simulink model "SingleTrack"  (R2019b)
settings: Solver=ode1  StartTime=0  StopTime=250  FixedStep=1.0000000000000000e-003  RelTol=1e-3
InitFcn:
  | sampleTime = str2double(get_param(bdroot, 'FixedStep'));
undefined symbols (not defined in the file or in its folder): AccPedalPos, BrakePedalPos, BrakeSwitch, DiscIntNeverNeededParam, DYNA4, EngSpd, IgnitionSwitch, InitialGear, InitialSpeed, IntendedEngTrq, LeftIndicator, MainBrakePress, MaxGear, MDL, MinGear, RefAcc, RefLane, RefLatPos, RefPath, RefPathCurv, RefSpd, RefSpdPreview, RefSpdRetrospect, RightIndicator, SteeringWheelAng, SteeringWheelTrq, UserDefinedRefValue, vm_const
libraries: UtilitiesLibrary x31, simulink x18, WheelSystemModules x13, LongitudinalControllerModules x13, LateralControllerModules x7, AnimationBusselectorModules x5, EnvironmentModules x5, BasicEngineControlModules x5, MiscellaneousControlModules x5, Animation3Modules x4, AuxiliariesModules x4, ReducedTireModules x4
(part 20 of 32)

== system SingleTrack/Vehicle/WheelSystem/FrontLeftWheelSystem/Tire ==
  fromCTRL : Inport
  fromChassis : Inport  Port=2
  fromWheel : Inport  Port=3
  Contact : WheelSystemModules/Contact  Tag=vedynaContactMask  local_comp_inst=1  system_comp_inst=1  sample_time=-1
  DynaComponentInfo : Subsystem  Tag=DynaComponentInfo
      mask init:
      | data= get_param(gcb, 'UserData');
      settings: OpenFcn=DYNA4.ModelHandling.Component.ShowEditComponentInformationDialog(gcb);
      mask Display: disp(['Type = ', data.type, '\nGroup = ', data.group, '\nName = ', data.name])
  Ground{1..3,5} (4 alike) : Ground
  InputFromCTRL : Subsystem  Tag=TESIS DYNAware Interface Block  mask{NeedsUpdate=off, SignalInfo=|}
      mask SignalInfo=|
      | {
      |   "Version": "4.6",
      |   "MuxedOutputBusName": "output",
      |   "MuxedInputBusName": "fromCTRL",
      |   "MuxedInputSelected": true,
      |   "MuxedOutputSelected": false,
      |   "SignalData": [
      |     {
      |       "initialValue": "0.0",
      |       "name": "AddRoadElev[m]",
      |       "comment": "",
      |       "minString": "",
      |       "maxString": "",
      |       "width": 1,
      |       "dataType": 0,
      |       "signalType": 0,
      |       "createSignal": false,
      |       "outputName": "AddRoadElev[m]",
      |       "generateSignalAccessBlock": false,
      |       "accessId": "$(parentId).$(blockName).$(outputName)"
      |     },
      |     {
      |       "initialValue": "0.0",
      |       "name": "RoadFrictionScaling[0_2]",
      |       "comment": "",
      |       "minString": "",
      |       "maxString": "",
      |       "width": 1,
      |       "dataType": 0,
      |       "signalType": 0,
      |       "createSignal": false,
      |       "outputName": "RoadFrictionScaling[0_2]",
      |       "generateSignalAccessBlock": false,
      |       "accessId": "$(parentId).$(blockName).$(outputName)"
      |     },
      |     {
      |       "initialValue": "0.0",
      |       "name": "AddLongRoadSlope[-]",
      |       "comment": "",
      |       "minString": "",
      |       "maxString": "",
      |       "width": 1,
      |       "dataType": 0,
      |       "signalType": 0,
      |       "createSignal": false,
      |       "outputName": "AddLongRoadSlope[-]",
      |       "generateSignalAccessBlock": false,
      |       "accessId": "$(parentId).$(blockName).$(outputName)"
      |     },
      |     {
      |       "initialValue": "0.0",
      |       "name": "AddLatRoadSlope[-]",
      |       "comment": "",
      |       "minString": "",
      |       "maxString": "",
      |       "width": 1,
      |       "dataType": 0,
      |       "signalType": 0,
      |       "createSignal": false,
      |       "outputName": "AddLatRoadSlope[-]",
      |       "generateSignalAccessBlock": false,
      |       "accessId": "$(parentId).$(blockName).$(outputName)"
      |     },
      |     {
      |       "initialValue": "0.0",
      |       "name": "LocalRoadSysSwitch[0;1]",
      |       "comment": "",
      |       "minString": "",
      |       "maxString": "",
      |       "width": 1,
      |       "dataType": 0,
      |       "signalType": 0,
      |       "createSignal": false,
      |       "outputName": "LocalRoadSysSwitch[0;1]",
      |       "generateSignalAccessBlock": false,
      |       "accessId": "$(parentId).$(blockName).$(outputName)"
      |     }
      |   ]
      | }
      mask prompts: NeedsUpdate "Specify, if subsystem content needs to be updated"; SignalInfo "Signal Info (json)"
      mask help: DYNA4 Interface Block Version 4.6
      mask init:
      | blockName = get_param(gcbh, 'Name');
      | parentId = DYNA4.ModelHandling.AccessID.getFromHierarchy(gcbh);
      | TD.InterfaceBlock.ModelCallbacks.GenerateContent(gcb);
      settings: DeleteFcn=TD.InterfaceBlock.ModelCallbacks.CloseGUI( gcbh );  NameChangeFcn=TD.InterfaceBlock.ModelCallbacks.BlockRenamedHandler(gcbh);  OpenFcn=TD.InterfaceBlock.ModelCallbacks.OpenGUI( gcbh );  CloseFcn=TD.InterfaceBlock.ModelCallbacks.CloseGUI( gcbh );
      mask Display:
      | image('InterfaceBlock.png','center');
      | port_label('input',1, 'fromCTRL');
      | port_label('output',1, 'AddRoadElev[m]');
      | port_label('output',2, 'RoadFrictionScaling[0_2]');
      | port_label('output',3, 'AddLongRoadSlope[-]');
      | port_label('output',4, 'AddLatRoadSlope[-]');
      | port_label('output',5, 'LocalRoadSysSwitch[0;1]');
  InputFromChassis : Subsystem  Tag=TESIS DYNAware Interface Block  mask{NeedsUpdate=off, SignalInfo=|}
      mask SignalInfo=|
      | {
      |   "Version": "4.6",
      |   "MuxedOutputBusName": "output",
      |   "MuxedInputBusName": "fromChassis",
      |   "MuxedInputSelected": true,
      |   "MuxedOutputSelected": false,
      |   "SignalData": [
      |     {
      |       "initialValue": "0.0",
      |       "name": "VehicleBody.PosAxleSys(WorldSys)",
      |       "comment": "",
      |       "minString": "",
      |       "maxString": "",
      |       "width": -1,
      |       "dataType": 0,
      |       "signalType": 0,
      |       "createSignal": false,
      |       "outputName": "PosAxleSys(WorldSys)",
      |       "generateSignalAccessBlock": false,
      |       "accessId": "$(parentId).$(blockName).$(outputName)"
      |     },
      |     {
      |       "initialValue": "0.0",
      |       "name": "VehicleBody.RotMatrix(WorldSys)[-]",
      |       "comment": "",
      |       "minString": "",
      |       "maxString": "",
      |       "width": 9,
      |       "dataType": 0,
      |       "signalType": 0,
      |       "createSignal": false,
      |       "outputName": "RotMatrix(WorldSys)[-]",
      |       "generateSignalAccessBlock": false,
      |       "accessId": "$(parentId).$(blockName).$(outputName)"
      |     },
      |     {
      |       "initialValue": "0.0",
      |       "name": "WheelSystem.WheelRotAxis(VehSys)[-]",
      |       "comment": "",
      |       "minString": "",
      |       "maxString": "",
      |       "width": 3,
      |       "dataType": 0,
      |       "signalType": 0,
      |       "createSignal": false,
      |       "outputName": "WheelRotAxis(VehSys)[-]",
      |       "generateSignalAccessBlock": false,
      |       "accessId": "$(parentId).$(blockName).$(outputName)"
      |     },
      |     {
      |       "initialValue": "0.0",
      |       "name": "WheelSystem.TirePos(AxleSys)[m]",
      |       "comment": "",
      |       "minString": "",
      |       "maxString": "",
      |       "width": -1,
      |       "dataType": 0,
      |       "signalType": 0,
      |       "createSignal": false,
      |       "outputName": "TirePos(AxleSys)[m]",
      |       "generateSignalAccessBlock": false,
      |       "accessId": "$(parentId).$(blockName).$(outputName)"
      |     },
      |     {
      |       "initialValue": "0.0",
      |       "name": "WheelSystem.TireVel_wrt_WorldSys(VehSys)[m/s]",
      |       "comment": "",
      |       "minString": "",
      |       "maxString": "",
      |       "width": 3,
      |       "dataType": 0,
      |       "signalType": 0,
      |       "createSignal": false,
      |       "outputName": "TireVel_wrt_WorldSys(VehSys)[m/s]",
      |       "generateSignalAccessBlock": false,
      |       "accessId": "$(parentId).$(blockName).$(outputName)"
      |     },
      |     {
      |       "initialValue": "0.0",
      |       "name": "WheelSystem.WheelRotVel_wrt_WorldSys(VehSys)[rad/s]",
      |       "comment": "",
      |       "minString": "",
      |       "maxString": "",
      |       "width": 3,
      |       "dataType": 0,
      |       "signalType": 0,
      |       "createSignal": false,
      |       "outputName": "WheelRotVel_wrt_WorldSys(VehSys)[rad/s]",
      |       "generateSignalAccessBlock": false,
      |       "accessId": "$(parentId).$(blockName).$(outputName)"
      |     },
      |     {
      |       "initialValue": "0.0",
      |       "name": "VehicleBody.Vel_wrt_WorldSys(VehSys)[m/s]",
      |       "comment": "",
      |       "minString": "",
      |       "maxString": "",
      |       "width": 3,
      |       "dataType": 0,
      |       "signalType": 0,
      |       "createSignal": false,
      |       "outputName": "Vel_wrt_WorldSys(VehSys)[m/s]",
      |       "generateSignalAccessBlock": false,
      |       "accessId": "$(parentId).$(blockName).$(outputName)"
      |     },
      |     {
      |       "initialValue": "0.0",
      |       "name": "WheelSystem.WheelRotMatrix(WorldSys)[-]",
      |       "comment": "",
      |       "minString": "",
      |       "maxString": "",
      |       "width": 9,
      |       "dataType": 0,
      |       "signalType": 0,
      |       "createSignal": false,
      |       "outputName": "WheelRotMatrix(WorldSys)[-]",
      |       "generateSignalAccessBlock": false,
      |       "accessId": "$(parentId).$(blockName).$(outputName)"
      |     },
      |     {
      |       "initialValue": "0.0",
      |       "name": "WheelSystem.TireDefl[m]",
      |       "comment": "",
      |       "minString": "",
      |       "maxString": "",
      |       "width": 1,
      |       "dataType": 0,
      |       "signalType": 0,
      |       "createSignal": false,
      |       "outputName": "TireDefl[m]",
      |       "generateSignalAccessBlock": false,
      |       "accessId": "$(parentId).$(blockName).$(outputName)"
      |     }
      |   ]
      | }
      mask prompts: NeedsUpdate "Specify, if subsystem content needs to be updated"; SignalInfo "Signal Info (json)"
      mask help: DYNA4 Interface Block Version 4.6
      mask init:
      | blockName = get_param(gcbh, 'Name');
      | parentId = DYNA4.ModelHandling.AccessID.getFromHierarchy(gcbh);
      | TD.InterfaceBlock.ModelCallbacks.GenerateContent(gcb);
      settings: DeleteFcn=TD.InterfaceBlock.ModelCallbacks.CloseGUI( gcbh );  NameChangeFcn=TD.InterfaceBlock.ModelCallbacks.BlockRenamedHandler(gcbh);  OpenFcn=TD.InterfaceBlock.ModelCallbacks.OpenGUI( gcbh );  CloseFcn=TD.InterfaceBlock.ModelCallbacks.CloseGUI( gcbh );
      mask Display:
      | image('InterfaceBlock.png','center');
      | port_label('input',1, 'fromChassis');
      | port_label('output',1, 'PosAxleSys(WorldSys)');
      | port_label('output',2, 'RotMatrix(WorldSys)[-]');
      | port_label('output',3, 'WheelRotAxis(VehSys)[-]');
      | port_label('output',4, 'TirePos(AxleSys)[m]');
      | port_label('output',5, 'TireVel_wrt_WorldSys(VehSys)[m/s]');
      | port_label('output',6, 'WheelRotVel_wrt_WorldSys(VehSys)[rad/s]');
      | port_label('output',7, 'Vel_wrt_WorldSys(VehSys)[m/s]');
      | port_label('output',8, 'WheelRotMatrix(WorldSys)[-]');
      | port_label('output',9, 'TireDefl[m]');
  InputFromWheel : Subsystem  Tag=TESIS DYNAware Interface Block  mask{NeedsUpdate=off, SignalInfo=|}
      mask SignalInfo=|
      | {
      |   "Version": "4.6",
      |   "MuxedOutputBusName": "fromWheel",
      |   "MuxedInputBusName": "fromWheel",
      |   "MuxedInputSelected": true,
      |   "MuxedOutputSelected": false,
      |   "SignalData": [
      |     {
      |       "initialValue": "0.0",
      |       "name": "RotSpd[rad/s]",
      |       "comment": "",
      |       "minString": "",
      |       "maxString": "",
      |       "width": 1,
      |       "dataType": 0,
      |       "signalType": 0,
      |       "createSignal": false,
      |       "outputName": "RotSpd[rad/s]",
      |       "generateSignalAccessBlock": false,
      |       "accessId": "$(parentId).$(blockName).$(outputName)"
      |     },
      |     {
      |       "initialValue": "0.0",
      |       "name": "BlockingState[0;1]",
      |       "comment": "",
      |       "minString": "",
      |       "maxString": "",
      |       "width": 1,
      |       "dataType": 0,
      |       "signalType": 0,
      |       "createSignal": false,
      |       "outputName": "BlockingState[0;1]",
      |       "generateSignalAccessBlock": false,
      |       "accessId": "$(parentId).$(blockName).$(outputName)"
      |     }
      |   ]
      | }
      mask prompts: NeedsUpdate "Specify, if subsystem content needs to be updated"; SignalInfo "Signal Info (json)"
      mask help: DYNA4 Interface Block Version 4.6
      mask init:
      | blockName = get_param(gcbh, 'Name');
      | parentId = DYNA4.ModelHandling.AccessID.getFromHierarchy(gcbh);
      | TD.InterfaceBlock.ModelCallbacks.GenerateContent(gcb);
      settings: DeleteFcn=TD.InterfaceBlock.ModelCallbacks.CloseGUI( gcbh );  NameChangeFcn=TD.InterfaceBlock.ModelCallbacks.BlockRenamedHandler(gcbh);  OpenFcn=TD.InterfaceBlock.ModelCallbacks.OpenGUI( gcbh );  CloseFcn=TD.InterfaceBlock.ModelCallbacks.CloseGUI( gcbh );
      mask Display:
      | image('InterfaceBlock.png','center');
      | port_label('input',1, 'fromWheel');
      | port_label('output',1, 'RotSpd[rad/s]');
      | port_label('output',2, 'BlockingState[0;1]');
  Memory1 : Memory  InheritSampleTime=on
  TabledTireForces : ReducedTireModules/TabledTireForces  Tag=vedynaTabledConsumptionMask  DATA_NODE=MDL.Vehicle.WheelSystem.FrontLeft.Tire.TabledTireForces  UnloadedRadius=MDL.Vehicle.WheelSystem.FrontLeft.Tire.TabledTireForces.UnloadedRadius  WidthToRadiusRatio=MDL.Vehicle.WheelSystem.FrontLeft.Tire.TabledTireForces.WidthToRadiusRatio  HeightToRadiusRatio=MDL.Vehicle.WheelSystem.FrontLeft.Tire.TabledTireForces.HeightToRadiusRatio  RefLoad=MDL.Vehicle.WheelSystem.FrontLeft.Tire.TabledTireForces.RefLoad  LongFrcCurve=MDL.Vehicle.WheelSystem.FrontLeft.Tire.TabledTireForces.LongFrcCurve  LatFrcCurve=MDL.Vehicle.WheelSystem.FrontLeft.Tire.TabledTireForces.LatFrcCurve  RollResistance=MDL.Vehicle.WheelSystem.FrontLeft.Tire.TabledTireForces.RollResistCoeff  VertStiff=MDL.Vehicle.WheelSystem.FrontLeft.Tire.TabledTireForces.VertStiff
  Tire Output : Subsystem  Tag=TESIS DYNAware Interface Block  mask{NeedsUpdate=off, SignalInfo=|}
      mask SignalInfo=|
      | {
      |   "Version": "4.6",
      |   "MuxedOutputBusName": "Tire",
      |   "MuxedInputBusName": "input",
      |   "MuxedInputSelected": false,
      |   "MuxedOutputSelected": true,
      |   "SignalData": [
      |     {
      |       "initialValue": "0.0",
      |       "name": "ContactPointPos_wrt_WheelCenter(WorldSys)[m]",
      |       "comment": "",
      |       "minString": "",
      |       "maxString": "",
      |       "width": 3,
      |       "dataType": 0,
      |       "signalType": 0,
      |       "createSignal": false,
      |       "outputName": "ContactPointPos_wrt_WheelCenter(WorldSys)[m]",
      |       "generateSignalAccessBlock": false,
      |       "accessId": "$(parentId).$(blockName).$(outputName)"
      |     },
      |     {
      |       "initialValue": "0.0",
      |       "name": "CamberAng(ContactSys)[rad]",
      |       "comment": "",
      |       "minString": "",
      |       "maxString": "",
      |       "width": 1,
      |       "dataType": 0,
      |       "signalType": 0,
      |       "createSignal": false,
      |       "outputName": "CamberAng(ContactSys)[rad]",
      |       "generateSignalAccessBlock": false,
      |       "accessId": "$(parentId).$(blockName).$(outputName)"
      |     },
      |     {
      |       "initialValue": "0.0",
      |       "name": "TireDefl[m]",
      |       "comment": "",
      |       "minString": "",
      |       "maxString": "",
      |       "width": 1,
      |       "dataType": 0,
      |       "signalType": 0,
      |       "createSignal": false,
      |       "outputName": "TireDefl[m]",
      |       "generateSignalAccessBlock": false,
      |       "accessId": "$(parentId).$(blockName).$(outputName)"
      |     },
      |     {
      |       "initialValue": "0.0",
      |       "name": "TireDeflSpd[m/s]",
      |       "comment": "",
      |       "minString": "",
      |       "maxString": "",
      |       "width": 1,
      |       "dataType": 0,
      |       "signalType": 0,
      |       "createSignal": false,
      |       "outputName": "TireDeflSpd[m/s]",
      |       "generateSignalAccessBlock": false,
      |       "accessId": "$(parentId).$(blockName).$(outputName)"
      |     },
      |     {
      |       "initialValue": "0.0",
      |       "name": "LongSpd(ContactSys)[m/s]",
      |       "comment": "",
      |       "minString": "",
      |       "maxString": "",
      |       "width": 1,
      |       "dataType": 0,
      |       "signalType": 0,
      |       "createSignal": false,
      |       "outputName": "LongSpd(ContactSys)[m/s]",
      |       "generateSignalAccessBlock": false,
      |       "accessId": "$(parentId).$(blockName).$(outputName)"
      |     },
      |     {
      |       "initialValue": "0.0",
      |       "name": "LatSpd(ContactSys)[m/s]",
      |       "comment": "",
      |       "minString": "",
      |       "maxString": "",
      |       "width": 1,
      |       "dataType": 0,
      |       "signalType": 0,
      |       "createSignal": false,
      |       "outputName": "LatSpd(ContactSys)[m/s]",
      |       "generateSignalAccessBlock": false,
      |       "accessId": "$(parentId).$(blockName).$(outputName)"
      |     },
      |     {
      |       "initialValue": "0.0",
      |       "name": "BoreSpd(ContactSys)[rad/s]",
      |       "comment": "",
      |       "minString": "",
      |       "maxString": "",
      |       "width": 1,
      |       "dataType": 0,
      |       "signalType": 0,
      |       "createSignal": false,
      |       "outputName": "BoreSpd(ContactSys)[rad/s]",
      |       "generateSignalAccessBlock": false,
      |       "accessId": "$(parentId).$(blockName).$(outputName)"
      |     },
      |     {
      |       "initialValue": "0.0",
      |       "name": "LongFrcLeverArm_wrt_WheelRotAxis[m]",
      |       "comment": "",
      |       "minString": "",
      |       "maxString": "",
      |       "width": 1,
      |       "dataType": 0,
      |       "signalType": 0,
      |       "createSignal": false,
      |       "outputName": "LongFrcLeverArm_wrt_WheelRotAxis[m]",
      |       "generateSignalAccessBlock": false,
      |       "accessId": "$(parentId).$(blockName).$(outputName)"
      |     },
      |     {
      |       "initialValue": "0.0",
      |       "name": "LongUnitVector(WorldSys)[-]",
      |       "comment": "",
      |       "minString": "",
      |       "maxString": "",
      |       "width": 3,
      |       "dataType": 0,
      |       "signalType": 0,
      |       "createSignal": false,
      |       "outputName": "LongUnitVector(WorldSys)[-]",
      |       "generateSignalAccessBlock": false,
      |       "accessId": "$(parentId).$(blockName).$(outputName)"
      |     },
      |     {
      |       "initialValue": "0.0",
      |       "name": "LatUnitVector(WorldSys)[-]",
      |       "comment": "",
      |       "minString": "",
      |       "maxString": "",
      |       "width": 3,
      |       "dataType": 0,
      |       "signalType": 0,
      |       "createSignal": false,
      |       "outputName": "LatUnitVector(WorldSys)[-]",
      |       "generateSignalAccessBlock": false,
      |       "accessId": "$(parentId).$(blockName).$(outputName)"
      |     },
      |     {
      |       "initialValue": "0.0",
      |       "name": "RoadNormalVector(WorldSys)[-]",
      |       "comment": "",
      |       "minString": "",
      |       "maxString": "",
      |       "width": 3,
      |       "dataType": 0,
      |       "signalType": 0,
      |       "createSignal": false,
      |       "outputName": "RoadNormalVector(WorldSys)[-]",
      |       "generateSignalAccessBlock": false,
      |       "accessId": "$(parentId).$(blockName).$(outputName)"
      |     },
      |     {
      |       "initialValue": "0.0",
      |       "name": "RoadType[-]",
      |       "comment": "",
      |       "minString": "",
      |       "maxString": "",
      |       "width": 1,
      |       "dataType": 0,
      |       "signalType": 0,
      |       "createSignal": false,
      |       "outputName": "RoadType[-]",
      |       "generateSignalAccessBlock": false,
      |       "accessId": "$(parentId).$(blockName).$(outputName)"
      |     },
      |     {
      |       "initialValue": "0.0",
      |       "name": "RoadFrictionScalingCoeff[-]",
      |       "comment": "",
      |       "minString": "",
      |       "maxString": "",
      |       "width": 1,
      |       "dataType": 0,
      |       "signalType": 0,
      |       "createSignal": false,
      |       "outputName": "RoadFrictionScalingCoeff[-]",
      |       "generateSignalAccessBlock": false,
      |       "accessId": "$(parentId).$(blockName).$(outputName)"
      |     },
      |     {
      |       "initialValue": "0.0",
      |       "name": "ContactPointPos(WorldSys)[m]",
      |       "comment": "",
      |       "minString": "",
      |       "maxString": "",
      |       "width": 3,
      |       "dataType": 0,
      |       "signalType": 0,
      |       "createSignal": false,
      |       "outputName": "ContactPointPos(WorldSys)[m]",
      |       "generateSignalAccessBlock": false,
      |       "accessId": "$(parentId).$(blockName).$(outputName)"
      |     },
      |     {
      |       "initialValue": "0.0",
      |       "name": "RoadSlope(WorldSys)[-]",
      |       "comment": "",
      |       "minString": "",
      |       "maxString": "",
      |       "width": 1,
      |       "dataType": 0,
      |       "signalType": 0,
      |       "createSignal": false,
      |       "outputName": "RoadSlope(WorldSys)[-]",
      |       "generateSignalAccessBlock": false,
      |       "accessId": "$(parentId).$(blockName).$(outputName)"
      |     },
      |     {
      |       "initialValue": "0.0",
      |       "name": "RoadIncl(WorldSys)[-]",
      |       "comment": "",
      |       "minString": "",
      |       "maxString": "",
      |       "width": 1,
      |       "dataType": 0,
      |       "signalType": 0,
      |       "createSignal": false,
      |       "outputName": "RoadIncl(WorldSys)[-]",
      |       "generateSignalAccessBlock": false,
      |       "accessId": "$(parentId).$(blockName).$(outputName)"
      |     },
      |     {
      |       "initialValue": "0.0",
      |       "name": "LocalContactPoints(WorldSys)[m]",
      |       "comment": "",
      |       "minString": "",
      |       "maxString": "",
      |       "width": 12,
      |       "dataType": 0,
      |       "signalType": 0,
      |       "createSignal": false,
      |       "outputName": "LocalContactPoints(WorldSys)[m]",
      |       "generateSignalAccessBlock": false,
      |       "accessId": "$(parentId).$(blockName).$(outputName)"
      |     },
      |     {
      |       "initialValue": "0.0",
      |       "name": "NumberOfLocalContactPoints[-]",
      |       "comment": "",
      |       "minString": "",
      |       "maxString": "",
      |       "width": 1,
      |       "dataType": 0,
      |       "signalType": 0,
      |       "createSignal": false,
      |       "outputName": "NumberOfLocalContactPoints[-]",
      |       "generateSignalAccessBlock": false,
      |       "accessId": "$(parentId).$(blockName).$(outputName)"
      |     },
      |     {
      |       "initialValue": "0.0",
      |       "name": "WheelCenterFrc(VehSys)[N]",
      |       "comment": "",
      |       "minString": "",
      |       "maxString": "",
      |       "width": 3,
      |       "dataType": 0,
      |       "signalType": 0,
      |       "createSignal": false,
      |       "outputName": "WheelCenterFrc(VehSys)[N]",
      |       "generateSignalAccessBlock": false,
      |       "accessId": "$(parentId).$(blockName).$(outputName)"
      |     },
      |     {
      |       "initialValue": "0.0",
      |       "name": "CircumferentialTrq_wrt_WheelRotAxis[Nm]",
      |       "comment": "",
      |       "minString": "",
      |       "maxString": "",
      |       "width": 1,
      |       "dataType": 0,
      |       "signalType": 0,
      |       "createSignal": false,
      |       "outputName": "CircumferentialTrq_wrt_WheelRotAxis[Nm]",
      |       "generateSignalAccessBlock": false,
      |       "accessId": "$(parentId).$(blockName).$(outputName)"
      |     },
      |     {
      |       "initialValue": "0.0",
      |       "name": "MaxRollResistTrq[Nm]",
      |       "comment": "",
      |       "minString": "",
      |       "maxString": "",
      |       "width": 1,
      |       "dataType": 0,
      |       "signalType": 0,
      |       "createSignal": false,
      |       "outputName": "MaxRollResistTrq[Nm]",
      |       "generateSignalAccessBlock": false,
      |       "accessId": "$(parentId).$(blockName).$(outputName)"
      |     },
      |     {
      |       "initialValue": "0.0",
      |       "name": "VertStiff[N/m]",
      |       "comment": "",
      |       "minString": "",
      |       "maxString": "",
      |       "width": 1,
      |       "dataType": 0,
      |       "signalType": 0,
      |       "createSignal": false,
      |       "outputName": "VertStiff[N/m]",
      |       "generateSignalAccessBlock": false,
      |       "accessId": "$(parentId).$(blockName).$(outputName)"
      |     },
      |     {
      |       "initialValue": "0.0",
      |       "name": "UnloadedRadius[m]",
      |       "comment": "",
      |       "minString": "",
      |       "maxString": "",
      |       "width": 1,
      |       "dataType": 0,
      |       "signalType": 0,
      |       "createSignal": false,
      |       "outputName": "UnloadedRadius[m]",
      |       "generateSignalAccessBlock": false,
      |       "accessId": "$(parentId).$(blockName).$(outputName)"
      |     },
      |     {
      |       "initialValue": "0.0",
      |       "name": "RimRadius[m]",
      |       "comment": "",
      |       "minString": "",
      |       "maxString": "",
      |       "width": 1,
      |       "dataType": 0,
      |       "signalType": 0,
      |       "createSignal": false,
      |       "outputName": "RimRadius[m]",
      |       "generateSignalAccessBlock": false,
      |       "accessId": "$(parentId).$(blockName).$(outputName)"
      |     },
      |     {
      |       "initialValue": "0.0",
      |       "name": "Width[m]",
      |       "comment": "",
      |       "minString": "",
      |       "maxString": "",
      |       "width": 1,
      |       "dataType": 0,
      |       "signalType": 0,
      |       "createSignal": false,
      |       "outputName": "Width[m]",
      |       "generateSignalAccessBlock": false,
      |       "accessId": "$(parentId).$(blockName).$(outputName)"
      |     },
      |     {
      |       "initialValue": "0.0",
      |       "name": "ContactPointFrc(ContactSys)[N]",
      |       "comment": "",
      |       "minString": "",
      |       "maxString": "",
      |       "width": 3,
      |       "dataType": 0,
      |       "signalType": 0,
      |       "createSignal": false,
      |       "outputName": "ContactPointFrc(ContactSys)[N]",
      |       "generateSignalAccessBlock": false,
      |       "accessId": "$(parentId).$(blockName).$(outputName)"
      |     },
      |     {
      |       "initialValue": "0.0",
      |       "name": "ContactPointTrq(ContactSys)[N]",
      |       "comment": "",
      |       "minString": "",
      |       "maxString": "",
      |       "width": 3,
      |       "dataType": 0,
      |       "signalType": 0,
      |       "createSignal": false,
      |       "outputName": "ContactPointTrq(ContactSys)[N]",
      |       "generateSignalAccessBlock": false,
      |       "accessId": "$(parentId).$(blockName).$(outputName)"
      |     },
      |     {
      |       "initialValue": "0.0",
      |       "name": "CorneringStiff[N]",
      |       "comment": "",
      |       "minString": "",
      |       "maxString": "",
      |       "width": 1,
      |       "dataType": 0,
      |       "signalType": 0,
      |       "createSignal": false,
      |       "outputName": "CorneringStiff[N]",
      |       "generateSignalAccessBlock": false,
      |       "accessId": "$(parentId).$(blockName).$(outputName)"
      |     },
      |     {
      |       "initialValue": "0.0",
      |       "name": "DynamicRadius[m]",
      |       "comment": "",
      |       "minString": "",
      |       "maxString": "",
      |       "width": 1,
      |       "dataType": 0,
      |       "signalType": 0,
      |       "createSignal": false,
      |       "outputName": "DynamicRadius[m]",
      |       "generateSignalAccessBlock": false,
      |       "accessId": "$(parentId).$(blockName).$(outputName)"
      |     },
      |     {
      |       "initialValue": "0.0",
      |       "name": "ContactPatchLength[m]",
      |       "comment": "",
      |       "minString": "",
      |       "maxString": "",
      |       "width": 1,
      |       "dataType": 0,
      |       "signalType": 0,
      |       "createSignal": false,
      |       "outputName": "ContactPatchLength[m]",
      |       "generateSignalAccessBlock": false,
      |       "accessId": "$(parentId).$(blockName).$(outputName)"
      |     },
      |     {
      |       "initialValue": "0.0",
      |       "name": "ContactPatchWidth[m]",
      |       "comment": "",
      |       "minString": "",
      |       "maxString": "",
      |       "width": 1,
      |       "dataType": 0,
      |       "signalType": 0,
      |       "createSignal": false,
      |       "outputName": "ContactPatchWidth[m]",
      |       "generateSignalAccessBlock": false,
      |       "accessId": "$(parentId).$(blockName).$(outputName)"
      |     }
      |   ]
      | }
      mask prompts: NeedsUpdate "Specify, if subsystem content needs to be updated"; SignalInfo "Signal Info (json)"
      mask help: DYNA4 Interface Block Version 4.6
      mask init:
      | blockName = get_param(gcbh, 'Name');
      | parentId = DYNA4.ModelHandling.AccessID.getFromHierarchy(gcbh);
      | TD.InterfaceBlock.ModelCallbacks.GenerateContent(gcb);
      settings: DeleteFcn=TD.InterfaceBlock.ModelCallbacks.CloseGUI( gcbh );  NameChangeFcn=TD.InterfaceBlock.ModelCallbacks.BlockRenamedHandler(gcbh);  OpenFcn=TD.InterfaceBlock.ModelCallbacks.OpenGUI( gcbh );  CloseFcn=TD.InterfaceBlock.ModelCallbacks.CloseGUI( gcbh );
      mask Display:
      | image('InterfaceBlock.png','center');
      | port_label('input',1, 'ContactPointPos_wrt_WheelCenter(WorldSys)[m]');
      | port_label('input',2, 'CamberAng(ContactSys)[rad]');
      | port_label('input',3, 'TireDefl[m]');
      | port_label('input',4, 'TireDeflSpd[m/s]');
      | port_label('input',5, 'LongSpd(ContactSys)[m/s]');
      | port_label('input',6, 'LatSpd(ContactSys)[m/s]');
      | port_label('input',7, 'BoreSpd(ContactSys)[rad/s]');
      | port_label('input',8, 'LongFrcLeverArm_wrt_WheelRotAxis[m]');
      | port_label('input',9, 'LongUnitVector(WorldSys)[-]');
      | port_label('input',10, 'LatUnitVector(WorldSys)[-]');
      | port_label('input',11, 'RoadNormalVector(WorldSys)[-]');
      | port_label('input',12, 'RoadType[-]');
      | port_label('input',13, 'RoadFrictionScalingCoeff[-]');
      | port_label('input',14, 'ContactPointPos(WorldSys)[m]');
      | port_label('input',15, 'RoadSlope(WorldSys)[-]');
      | port_label('input',16, 'RoadIncl(WorldSys)[-]');
      | port_label('input',17, 'LocalContactPoints(WorldSys)[m]');
      | port_label('input',18, 'NumberOfLocalContactPoints[-]');
      | port_label('input',19, 'WheelCenterFrc(VehSys)[N]');
      | port_label('input',20, 'CircumferentialTrq_wrt_WheelRotAxis[Nm]');
      | port_label('input',21, 'MaxRollResistTrq[Nm]');
      | port_label('input',22, 'VertStiff[N/m]');
      | port_label('input',23, 'UnloadedRadius[m]');
      | port_label('input',24, 'RimRadius[m]');
      | port_label('input',25, 'Width[m]');
      | port_label('input',26, 'ContactPointFrc(ContactSys)[N]');
      | port_label('input',27, 'ContactPointTrq(ContactSys)[N]');
      | port_label('input',28, 'CorneringStiff[N]');
      | port_label('input',29, 'DynamicRadius[m]');
      | port_label('input',30, 'ContactPatchLength[m]');
      | port_label('input',31, 'ContactPatchWidth[m]');
      | port_label('output',1, 'Tire');
  TraceMarker : UtilitiesLibrary/DYNA4 Trace Marker  Tag=DYNA4_TRACE_MARKER  SettingType=Standard  PrefixModelBlockID=on  PrefixRootSignalName=off  NamePattern='$(modelBlockID).$(rootSignalName)'
  Tire : Outport  VectorParamsAs1DForOutWhenUnconnected=off
  wires:
  InputFromWheel/1(RotSpd[rad/s]___UNIQUE_1) -> TabledTireForces/7, Contact/5
  TabledTireForces/9 -> Tire Output/28(CorneringStiff[N]___UNIQUE_1)
  TabledTireForces/8 -> Tire Output/26(ContactPointFrc(ContactSys)[N]___UNIQUE_1)
  Ground5/1 -> Contact/1
  Memory1/1 -> TabledTireForces/8
  TabledTireForces/7 -> Contact/4, Tire Output/25(Width[m]___UNIQUE_1)
  fromChassis/1 -> InputFromChassis/1(fromChassis)
  fromCTRL/1 -> InputFromCTRL/1(fromCTRL)
  InputFromCTRL/5(LocalRoadSysSwitch[0;1]___UNIQUE_1) -> Contact/16
  InputFromCTRL/4(AddLatRoadSlope[-]___UNIQUE_1) -> Contact/15
  InputFromCTRL/3(AddLongRoadSlope[-]___UNIQUE_1) -> Contact/14
  InputFromCTRL/2(RoadFrictionScaling[0_2]___UNIQUE_1) -> Contact/13
  InputFromCTRL/1(AddRoadElev[m]___UNIQUE_1) -> Contact/12
  InputFromChassis/6(WheelRotVel_wrt_WorldSys(VehSys)[rad/s]___UNIQUE_1) -> Contact/11
  InputFromChassis/5(TireVel_wrt_WorldSys(VehSys)[m/s]___UNIQUE_1) -> Contact/10
  InputFromChassis/3(WheelRotAxis(VehSys)[-]___UNIQUE_1) -> Contact/8
  InputFromChassis/2(RotMatrix(WorldSys)[-]___UNIQUE_1) -> Contact/7, TabledTireForces/4
  InputFromChassis/1(PosAxleSys(WorldSys)___UNIQUE_1) -> Contact/6
  Contact/16 -> Tire Output/16(RoadIncl(WorldSys)[-]___UNIQUE_1)
  Contact/15 -> Tire Output/15(RoadSlope(WorldSys)[-]___UNIQUE_1)
  Contact/14 -> Tire Output/14(ContactPointPos(WorldSys)[m]___UNIQUE_1)
  Contact/13 -> Tire Output/13(RoadFrictionScalingCoeff[-]___UNIQUE_1)
  Contact/12 -> Tire Output/12(RoadType[-]___UNIQUE_1)
  Contact/11 -> Tire Output/11(RoadNormalVector(WorldSys)[-]___UNIQUE_1)
  Contact/10 -> Tire Output/10(LatUnitVector(WorldSys)[-]___UNIQUE_1)
  Contact/9 -> Tire Output/9(LongUnitVector(WorldSys)[-]___UNIQUE_1)
  Contact/8 -> Tire Output/8(LongFrcLeverArm_wrt_WheelRotAxis[m]___UNIQUE_1)
  Contact/7 -> Tire Output/7(BoreSpd(ContactSys)[rad/s]___UNIQUE_1)
  Contact/6 -> TabledTireForces/2, Tire Output/6(LatSpd(ContactSys)[m/s]___UNIQUE_1)
  Contact/5 -> TabledTireForces/1, Tire Output/5(LongSpd(ContactSys)[m/s]___UNIQUE_1)
  Contact/4 -> Tire Output/4(TireDeflSpd[m/s]___UNIQUE_1)
  Contact/3 -> Tire Output/3(TireDefl[m]___UNIQUE_1)
  Contact/2 -> Tire Output/2(CamberAng(ContactSys)[rad]___UNIQUE_1)
  Contact/1 -> Tire Output/1(ContactPointPos_wrt_WheelCenter(WorldSys)[m]___UNIQUE_1)
  Tire Output/1(Tire___UNIQUE_1) -> Tire/1, TraceMarker/1
  fromWheel/1 -> InputFromWheel/1(fromWheel)
  TabledTireForces/2 -> Tire Output/20(CircumferentialTrq_wrt_WheelRotAxis[Nm]___UNIQUE_1)
  TabledTireForces/4 -> Tire Output/22(VertStiff[N/m]___UNIQUE_1)
  TabledTireForces/6 -> Contact/3, Tire Output/24(RimRadius[m]___UNIQUE_1)
  TabledTireForces/3 -> Tire Output/21(MaxRollResistTrq[Nm]___UNIQUE_1)
  TabledTireForces/1 -> Tire Output/19(WheelCenterFrc(VehSys)[N]___UNIQUE_1)
  InputFromChassis/7(Vel_wrt_WorldSys(VehSys)[m/s]___UNIQUE_1) -> TabledTireForces/5
  InputFromChassis/8(WheelRotMatrix(WorldSys)[-]___UNIQUE_1) -> TabledTireForces/6
  InputFromWheel/2(BlockingState[0;1]___UNIQUE_1) -> Memory1/1
  TabledTireForces/5 -> Contact/2, Tire Output/23(UnloadedRadius[m]___UNIQUE_1), Tire Output/29(DynamicRadius[m]___UNIQUE_1)
  InputFromChassis/9(TireDefl[m]___UNIQUE_1) -> TabledTireForces/3
  Contact/17 -> Tire Output/17(LocalContactPoints(WorldSys)[m]___UNIQUE_1)
  Contact/18 -> Tire Output/18(NumberOfLocalContactPoints[-]___UNIQUE_1)
  Ground1/1 -> Tire Output/30(ContactPatchLength[m]___UNIQUE_1)
  Ground2/1 -> Tire Output/27(ContactPointTrq(ContactSys)[N]___UNIQUE_1)
  Ground3/1 -> Tire Output/31(ContactPatchWidth[m]___UNIQUE_1)
  InputFromChassis/4(TirePos(AxleSys)[m]___UNIQUE_1) -> Contact/9

== system SingleTrack/Vehicle/WheelSystem/FrontLeftWheelSystem/WheelOutput ==
  DriveBrakeTrq_wrt_WheelRotAxis(VehSys)[Nm]___UNIQUE_1 : Inport  Description=|  PortDimensions=[3]
      | <name>DriveBrakeTrq_wrt_WheelRotAxis(VehSys)[Nm]</name>
      | <comment></comment>
  RotSpd[rad/s]___UNIQUE_1 : Inport  Description=|  Port=2  PortDimensions=[1]
      | <name>RotSpd[rad/s]</name>
      | <comment></comment>
  RotAcc[rad/s**2]___UNIQUE_1 : Inport  Description=|  Port=3  PortDimensions=[1]
      | <name>RotAcc[rad/s**2]</name>
      | <comment></comment>
  BlockingState[0;1]___UNIQUE_1 : Inport  Description=|  Port=4  PortDimensions=[1]
      | <name>BlockingState[0;1]</name>
      | <comment></comment>
  RotAng[rad]___UNIQUE_1 : Inport  Description=|  Port=5  PortDimensions=[1]
      | <name>RotAng[rad]</name>
      | <comment></comment>
  BrakeTrqPressRatio[m**3]___UNIQUE_1 : Inport  Description=|  Port=6  PortDimensions=[1]
      | <name>BrakeTrqPressRatio[m**3]</name>
      | <comment></comment>
  RotAxisInrt[kg*m**2]___UNIQUE_1 : Inport  Description=|  Port=7  PortDimensions=[1]
      | <name>RotAxisInrt[kg*m**2]</name>
      | <comment></comment>
  TotalResistanceTorque[Nm]___UNIQUE_1 : Inport  Description=|  Port=8  PortDimensions=[1]
      | <name>TotalResistanceTorque[Nm]</name>
      | <comment></comment>
  KinematicWheelActiveFlag[0;1]___UNIQUE_1 : Inport  Description=|  Port=9  PortDimensions=[1]
      | <name>KinematicWheelActiveFlag[0;1]</name>
      | <comment></comment>
  VehBodyReplacementInrt[kg*m**2]___UNIQUE_1 : Inport  Description=|  Port=10  PortDimensions=[1]
      | <name>VehBodyReplacementInrt[kg*m**2]</name>
      | <comment></comment>
  __TDD__Wheel.BlockingState[0;1] : Demux  Outputs=[1]
  __TDD__Wheel.BrakeTrqPressRatio[m**3] : Demux  Outputs=[1]
  __TDD__Wheel.DriveBrakeTrq_wrt_WheelRotAxis(VehSys)[Nm] : Demux  Outputs=[3]
  __TDD__Wheel.KinematicWheelActiveFlag[0;1] : Demux  Outputs=[1]
  __TDD__Wheel.RotAcc[rad/s**2] : Demux  Outputs=[1]
  __TDD__Wheel.RotAng[rad] : Demux  Outputs=[1]
  __TDD__Wheel.RotAxisInrt[kg*m**2] : Demux  Outputs=[1]
  __TDD__Wheel.RotSpd[rad/s] : Demux  Outputs=[1]
  __TDD__Wheel.TotalResistanceTorque[Nm] : Demux  Outputs=[1]
  __TDD__Wheel.VehBodyReplacementInrt[kg*m**2] : Demux  Outputs=[1]
  __TDO__Wheel : BusCreator  Inputs=10
  Wheel___UNIQUE_1 : Outport  Description=|  PortDimensions=[12]  VectorParamsAs1DForOutWhenUnconnected=off
      | <name>DriveBrakeTrq_wrt_WheelRotAxis(VehSys)[Nm]</name>
      | <comment></comment>
  wires:
  __TDO__Wheel/1 -> Wheel___UNIQUE_1/1  "Wheel"
  __TDD__Wheel.VehBodyReplacementInrt[kg*m**2]/1 -> __TDO__Wheel/10  "VehBodyReplacementInrt[kg*m**2]"
  VehBodyReplacementInrt[kg*m**2]___UNIQUE_1/1 -> __TDD__Wheel.VehBodyReplacementInrt[kg*m**2]/1
  __TDD__Wheel.KinematicWheelActiveFlag[0;1]/1 -> __TDO__Wheel/9  "KinematicWheelActiveFlag[0;1]"
  KinematicWheelActiveFlag[0;1]___UNIQUE_1/1 -> __TDD__Wheel.KinematicWheelActiveFlag[0;1]/1
  __TDD__Wheel.TotalResistanceTorque[Nm]/1 -> __TDO__Wheel/8  "TotalResistanceTorque[Nm]"
  TotalResistanceTorque[Nm]___UNIQUE_1/1 -> __TDD__Wheel.TotalResistanceTorque[Nm]/1
  __TDD__Wheel.RotAxisInrt[kg*m**2]/1 -> __TDO__Wheel/7  "RotAxisInrt[kg*m**2]"
  RotAxisInrt[kg*m**2]___UNIQUE_1/1 -> __TDD__Wheel.RotAxisInrt[kg*m**2]/1
  __TDD__Wheel.BrakeTrqPressRatio[m**3]/1 -> __TDO__Wheel/6  "BrakeTrqPressRatio[m**3]"
  BrakeTrqPressRatio[m**3]___UNIQUE_1/1 -> __TDD__Wheel.BrakeTrqPressRatio[m**3]/1
  __TDD__Wheel.RotAng[rad]/1 -> __TDO__Wheel/5  "RotAng[rad]"
  RotAng[rad]___UNIQUE_1/1 -> __TDD__Wheel.RotAng[rad]/1
  __TDD__Wheel.BlockingState[0;1]/1 -> __TDO__Wheel/4  "BlockingState[0;1]"
  BlockingState[0;1]___UNIQUE_1/1 -> __TDD__Wheel.BlockingState[0;1]/1
  __TDD__Wheel.RotAcc[rad/s**2]/1 -> __TDO__Wheel/3  "RotAcc[rad/s**2]"
  RotAcc[rad/s**2]___UNIQUE_1/1 -> __TDD__Wheel.RotAcc[rad/s**2]/1
  __TDD__Wheel.RotSpd[rad/s]/1 -> __TDO__Wheel/2  "RotSpd[rad/s]"
  RotSpd[rad/s]___UNIQUE_1/1 -> __TDD__Wheel.RotSpd[rad/s]/1
  __TDD__Wheel.DriveBrakeTrq_wrt_WheelRotAxis(VehSys)[Nm]/1 -> __TDO__Wheel/1  "DriveBrakeTrq_wrt_WheelRotAxis(VehSys)[Nm]"
  DriveBrakeTrq_wrt_WheelRotAxis(VehSys)[Nm]___UNIQUE_1/1 -> __TDD__Wheel.DriveBrakeTrq_wrt_WheelRotAxis(VehSys)[Nm]/1

== system SingleTrack/Vehicle/WheelSystem/FrontRightWheelSystem/DynaSystemInfo ==

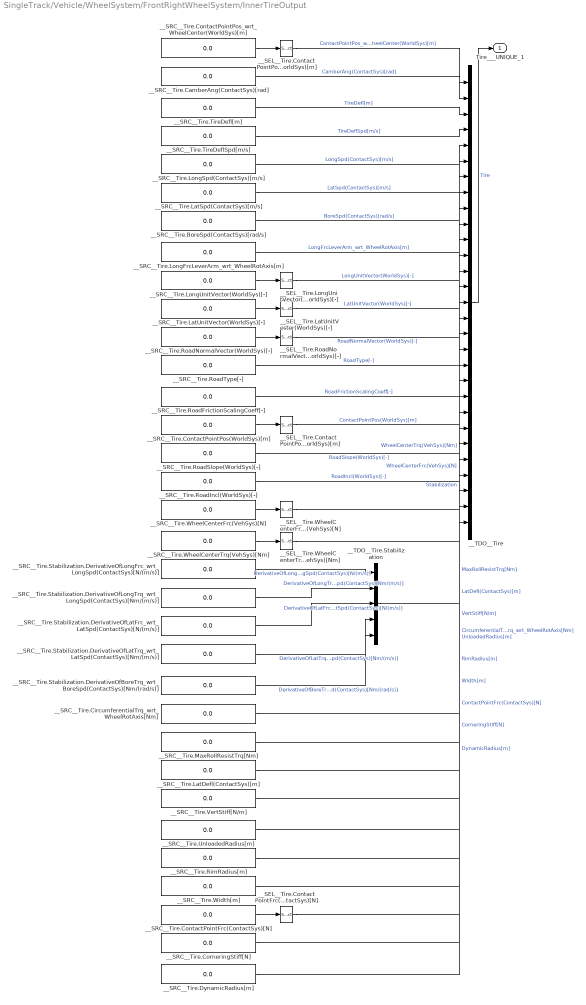
== system SingleTrack/Vehicle/WheelSystem/FrontRightWheelSystem/InnerTireOutput ==
  __SEL__Tire.ContactPointFrc(ContactSys)[N] : Selector  InputPortWidth=1  IndexOptions=Index vector (dialog)  Indices=ones(3, 1)  OutputSizes=1
  __SEL__Tire.ContactPointPos(WorldSys)[m] : Selector  InputPortWidth=1  IndexOptions=Index vector (dialog)  Indices=ones(3, 1)  OutputSizes=1
  __SEL__Tire.ContactPointPos_wrt_WheelCenter(WorldSys)[m] : Selector  InputPortWidth=1  IndexOptions=Index vector (dialog)  Indices=ones(3, 1)  OutputSizes=1
  __SEL__Tire.LatUnitVector(WorldSys)[-] : Selector  InputPortWidth=1  IndexOptions=Index vector (dialog)  Indices=ones(3, 1)  OutputSizes=1
  __SEL__Tire.LongUnitVector(WorldSys)[-] : Selector  InputPortWidth=1  IndexOptions=Index vector (dialog)  Indices=ones(3, 1)  OutputSizes=1
  __SEL__Tire.RoadNormalVector(WorldSys)[-] : Selector  InputPortWidth=1  IndexOptions=Index vector (dialog)  Indices=ones(3, 1)  OutputSizes=1
  __SEL__Tire.WheelCenterFrc(VehSys)[N] : Selector  InputPortWidth=1  IndexOptions=Index vector (dialog)  Indices=ones(3, 1)  OutputSizes=1
  __SEL__Tire.WheelCenterTrq(VehSys)[Nm] : Selector  InputPortWidth=1  IndexOptions=Index vector (dialog)  Indices=ones(3, 1)  OutputSizes=1
  __SRC__Tire.BoreSpd(ContactSys)[rad/s] : Constant  Value=0.0  OutDataTypeStr=Inherit: Inherit via back propagation
  __SRC__Tire.CamberAng(ContactSys)[rad] : Constant  Value=0.0  OutDataTypeStr=Inherit: Inherit via back propagation
  __SRC__Tire.CircumferentialTrq_wrt_WheelRotAxis[Nm] : Constant  Value=0.0  OutDataTypeStr=Inherit: Inherit via back propagation
  __SRC__Tire.ContactPointFrc(ContactSys)[N] : Constant  Value=0.0  OutDataTypeStr=Inherit: Inherit via back propagation
  __SRC__Tire.ContactPointPos(WorldSys)[m] : Constant  Value=0.0  OutDataTypeStr=Inherit: Inherit via back propagation
  __SRC__Tire.ContactPointPos_wrt_WheelCenter(WorldSys)[m] : Constant  Value=0.0  OutDataTypeStr=Inherit: Inherit via back propagation
  __SRC__Tire.CorneringStiff[N] : Constant  Value=0.0  OutDataTypeStr=Inherit: Inherit via back propagation
  __SRC__Tire.DynamicRadius[m] : Constant  Value=0.0  OutDataTypeStr=Inherit: Inherit via back propagation
  __SRC__Tire.LatDefl(ContactSys)[m] : Constant  Value=0.0  OutDataTypeStr=Inherit: Inherit via back propagation
  __SRC__Tire.LatSpd(ContactSys)[m/s] : Constant  Value=0.0  OutDataTypeStr=Inherit: Inherit via back propagation
  __SRC__Tire.LatUnitVector(WorldSys)[-] : Constant  Value=0.0  OutDataTypeStr=Inherit: Inherit via back propagation
  __SRC__Tire.LongFrcLeverArm_wrt_WheelRotAxis[m] : Constant  Value=0.0  OutDataTypeStr=Inherit: Inherit via back propagation
  __SRC__Tire.LongSpd(ContactSys)[m/s] : Constant  Value=0.0  OutDataTypeStr=Inherit: Inherit via back propagation
  __SRC__Tire.LongUnitVector(WorldSys)[-] : Constant  Value=0.0  OutDataTypeStr=Inherit: Inherit via back propagation
  __SRC__Tire.MaxRollResistTrq[Nm] : Constant  Value=0.0  OutDataTypeStr=Inherit: Inherit via back propagation
  __SRC__Tire.RimRadius[m] : Constant  Value=0.0  OutDataTypeStr=Inherit: Inherit via back propagation
  __SRC__Tire.RoadFrictionScalingCoeff[-] : Constant  Value=0.0  OutDataTypeStr=Inherit: Inherit via back propagation
  __SRC__Tire.RoadIncl(WorldSys)[-] : Constant  Value=0.0  OutDataTypeStr=Inherit: Inherit via back propagation
  __SRC__Tire.RoadNormalVector(WorldSys)[-] : Constant  Value=0.0  OutDataTypeStr=Inherit: Inherit via back propagation
  __SRC__Tire.RoadSlope(WorldSys)[-] : Constant  Value=0.0  OutDataTypeStr=Inherit: Inherit via back propagation
  __SRC__Tire.RoadType[-] : Constant  Value=0.0  OutDataTypeStr=Inherit: Inherit via back propagation
  __SRC__Tire.Stabilization.DerivativeOfBoreTrq_wrt_BoreSpd(ContactSys)[Nm/(rad/s)] : Constant  Value=0.0  OutDataTypeStr=Inherit: Inherit via back propagation
  __SRC__Tire.Stabilization.DerivativeOfLatFrc_wrt_LatSpd(ContactSys)[N/(m/s)] : Constant  Value=0.0  OutDataTypeStr=Inherit: Inherit via back propagation
  __SRC__Tire.Stabilization.DerivativeOfLatTrq_wrt_LatSpd(ContactSys)[Nm/(m/s)] : Constant  Value=0.0  OutDataTypeStr=Inherit: Inherit via back propagation
  __SRC__Tire.Stabilization.DerivativeOfLongFrc_wrt_LongSpd(ContactSys)[N/(m/s)] : Constant  Value=0.0  OutDataTypeStr=Inherit: Inherit via back propagation
  __SRC__Tire.Stabilization.DerivativeOfLongTrq_wrt_LongSpd(ContactSys)[Nm/(m/s)] : Constant  Value=0.0  OutDataTypeStr=Inherit: Inherit via back propagation
  __SRC__Tire.TireDeflSpd[m/s] : Constant  Value=0.0  OutDataTypeStr=Inherit: Inherit via back propagation
  __SRC__Tire.TireDefl[m] : Constant  Value=0.0  OutDataTypeStr=Inherit: Inherit via back propagation
  __SRC__Tire.UnloadedRadius[m] : Constant  Value=0.0  OutDataTypeStr=Inherit: Inherit via back propagation
  __SRC__Tire.VertStiff[N/m] : Constant  Value=0.0  OutDataTypeStr=Inherit: Inherit via back propagation
  __SRC__Tire.WheelCenterFrc(VehSys)[N] : Constant  Value=0.0  OutDataTypeStr=Inherit: Inherit via back propagation
  __SRC__Tire.WheelCenterTrq(VehSys)[Nm] : Constant  Value=0.0  OutDataTypeStr=Inherit: Inherit via back propagation
  __SRC__Tire.Width[m] : Constant  Value=0.0  OutDataTypeStr=Inherit: Inherit via back propagation
  __TDO__Tire : BusCreator  Inputs=29
  __TDO__Tire.Stabilization : BusCreator  Inputs=5
  Tire___UNIQUE_1 : Outport  Description=|  PortDimensions=[49]  VectorParamsAs1DForOutWhenUnconnected=off
      | <name></name>
      | <comment></comment>
  wires:
  __TDO__Tire/1 -> Tire___UNIQUE_1/1  "Tire"
  __SRC__Tire.DynamicRadius[m]/1 -> __TDO__Tire/29  "DynamicRadius[m]"
  __SRC__Tire.CorneringStiff[N]/1 -> __TDO__Tire/28  "CorneringStiff[N]"
  __SEL__Tire.ContactPointFrc(ContactSys)[N]/1 -> __TDO__Tire/27  "ContactPointFrc(ContactSys)[N]"
  __SRC__Tire.Width[m]/1 -> __TDO__Tire/26  "Width[m]"
  __SRC__Tire.RimRadius[m]/1 -> __TDO__Tire/25  "RimRadius[m]"
  __SRC__Tire.UnloadedRadius[m]/1 -> __TDO__Tire/24  "UnloadedRadius[m]"
  __SRC__Tire.VertStiff[N/m]/1 -> __TDO__Tire/23  "VertStiff[N/m]"
  __SRC__Tire.LatDefl(ContactSys)[m]/1 -> __TDO__Tire/22  "LatDefl(ContactSys)[m]"
  __SRC__Tire.MaxRollResistTrq[Nm]/1 -> __TDO__Tire/21  "MaxRollResistTrq[Nm]"
  __SRC__Tire.CircumferentialTrq_wrt_WheelRotAxis[Nm]/1 -> __TDO__Tire/20  "CircumferentialTrq_wrt_WheelRotAxis[Nm]"
  __SRC__Tire.Stabilization.DerivativeOfBoreTrq_wrt_BoreSpd(ContactSys)[Nm/(rad/s)]/1 -> __TDO__Tire.Stabilization/5  "DerivativeOfBoreTrq_wrt_BoreSpd(ContactSys)[Nm/(rad/s)]"
  __SRC__Tire.Stabilization.DerivativeOfLatTrq_wrt_LatSpd(ContactSys)[Nm/(m/s)]/1 -> __TDO__Tire.Stabilization/4  "DerivativeOfLatTrq_wrt_LatSpd(ContactSys)[Nm/(m/s)]"
  __SRC__Tire.Stabilization.DerivativeOfLatFrc_wrt_LatSpd(ContactSys)[N/(m/s)]/1 -> __TDO__Tire.Stabilization/3  "DerivativeOfLatFrc_wrt_LatSpd(ContactSys)[N/(m/s)]"
  __SRC__Tire.Stabilization.DerivativeOfLongTrq_wrt_LongSpd(ContactSys)[Nm/(m/s)]/1 -> __TDO__Tire.Stabilization/2  "DerivativeOfLongTrq_wrt_LongSpd(ContactSys)[Nm/(m/s)]"
  __TDO__Tire.Stabilization/1 -> __TDO__Tire/19  "Stabilization"
  __SRC__Tire.Stabilization.DerivativeOfLongFrc_wrt_LongSpd(ContactSys)[N/(m/s)]/1 -> __TDO__Tire.Stabilization/1  "DerivativeOfLongFrc_wrt_LongSpd(ContactSys)[N/(m/s)]"
  __SEL__Tire.WheelCenterTrq(VehSys)[Nm]/1 -> __TDO__Tire/18  "WheelCenterTrq(VehSys)[Nm]"
  __SEL__Tire.WheelCenterFrc(VehSys)[N]/1 -> __TDO__Tire/17  "WheelCenterFrc(VehSys)[N]"
  __SRC__Tire.RoadIncl(WorldSys)[-]/1 -> __TDO__Tire/16  "RoadIncl(WorldSys)[-]"
  __SRC__Tire.RoadSlope(WorldSys)[-]/1 -> __TDO__Tire/15  "RoadSlope(WorldSys)[-]"
  __SEL__Tire.ContactPointPos(WorldSys)[m]/1 -> __TDO__Tire/14  "ContactPointPos(WorldSys)[m]"
  __SRC__Tire.RoadFrictionScalingCoeff[-]/1 -> __TDO__Tire/13  "RoadFrictionScalingCoeff[-]"
  __SRC__Tire.RoadType[-]/1 -> __TDO__Tire/12  "RoadType[-]"
  __SEL__Tire.RoadNormalVector(WorldSys)[-]/1 -> __TDO__Tire/11  "RoadNormalVector(WorldSys)[-]"
  __SEL__Tire.LatUnitVector(WorldSys)[-]/1 -> __TDO__Tire/10  "LatUnitVector(WorldSys)[-]"
  __SEL__Tire.LongUnitVector(WorldSys)[-]/1 -> __TDO__Tire/9  "LongUnitVector(WorldSys)[-]"
  __SRC__Tire.LongFrcLeverArm_wrt_WheelRotAxis[m]/1 -> __TDO__Tire/8  "LongFrcLeverArm_wrt_WheelRotAxis[m]"
  __SRC__Tire.BoreSpd(ContactSys)[rad/s]/1 -> __TDO__Tire/7  "BoreSpd(ContactSys)[rad/s]"
  __SRC__Tire.LatSpd(ContactSys)[m/s]/1 -> __TDO__Tire/6  "LatSpd(ContactSys)[m/s]"
  __SRC__Tire.LongSpd(ContactSys)[m/s]/1 -> __TDO__Tire/5  "LongSpd(ContactSys)[m/s]"
  __SRC__Tire.TireDeflSpd[m/s]/1 -> __TDO__Tire/4  "TireDeflSpd[m/s]"
  __SRC__Tire.TireDefl[m]/1 -> __TDO__Tire/3  "TireDefl[m]"
  __SRC__Tire.CamberAng(ContactSys)[rad]/1 -> __TDO__Tire/2  "CamberAng(ContactSys)[rad]"
  __SEL__Tire.ContactPointPos_wrt_WheelCenter(WorldSys)[m]/1 -> __TDO__Tire/1  "ContactPointPos_wrt_WheelCenter(WorldSys)[m]"
  __SRC__Tire.ContactPointFrc(ContactSys)[N]/1 -> __SEL__Tire.ContactPointFrc(ContactSys)[N]/1
  __SRC__Tire.WheelCenterTrq(VehSys)[Nm]/1 -> __SEL__Tire.WheelCenterTrq(VehSys)[Nm]/1
  __SRC__Tire.WheelCenterFrc(VehSys)[N]/1 -> __SEL__Tire.WheelCenterFrc(VehSys)[N]/1
  __SRC__Tire.ContactPointPos(WorldSys)[m]/1 -> __SEL__Tire.ContactPointPos(WorldSys)[m]/1
  __SRC__Tire.RoadNormalVector(WorldSys)[-]/1 -> __SEL__Tire.RoadNormalVector(WorldSys)[-]/1
  __SRC__Tire.LatUnitVector(WorldSys)[-]/1 -> __SEL__Tire.LatUnitVector(WorldSys)[-]/1
  __SRC__Tire.LongUnitVector(WorldSys)[-]/1 -> __SEL__Tire.LongUnitVector(WorldSys)[-]/1
  __SRC__Tire.ContactPointPos_wrt_WheelCenter(WorldSys)[m]/1 -> __SEL__Tire.ContactPointPos_wrt_WheelCenter(WorldSys)[m]/1
